simulink model "mip_balance"  (R2017b)
settings: Solver=FixedStepDiscrete  StartTime=0.0  StopTime=inf  RelTol=1e-3  EnableMultiTasking=on
undefined symbols (not defined in the file): DiscIntNeverNeededParam
libraries: beaglebonebluelib x8, simulink_extras x1, simulink x1
settings Model: FPTRunName=Active  SimulationMode=external  ExtModeTrigDuration=2  Creator=The MathWorks, Inc.  LastModifiedBy=pthb3
settings SolverCC: PositivePriorityOrder=on
settings DataIOCC: LimitDataPoints=on  SaveFormat=Array
settings OptimizationCC: ExpressionDepthLimit=2147483647  LifeSpan=Inf  MaxStackSize=64
settings DebuggingCC: UnderspecifiedInitializationDetection=Classic  MergeDetectMultiDrivingBlocksExec=none  FcnCallInpInsideContextMsg=warning  AllowSymbolicDim=off  StateNameClashWarn=warning  SFUnexpectedBacktrackingDiag=warning  SFNoUnconditionalDefaultTransitionDiag=warning  SFExecutionAtInitializationDiag=none
settings HardwareCC: ProdBitPerPointer=32  ProdBitPerSizeT=32  ProdBitPerPtrDiffT=32  ProdLargestAtomicInteger=Long  ProdLargestAtomicFloat=Double  ProdWordSize=32  ProdHWDeviceType=ARM Compatible->ARM Cortex  UseEmbeddedCoderFeatures=off
settings ModelReferenceCC: PropagateSignalLabelsOutOfModel=off
settings RTWCC: SystemTargetFile=ert.tlc  HardwareBoard=BeagleBone Blue  TemplateMakefile=ert_default_tmf  RTWVerbose=off  Toolchain=GNU GCC BeagleBone Blue
settings CodeAppCC: StateflowObjectComments=on
settings ERTTargetCC: MultiwordLength=2048  ERTCustomFileBanners=off  SupportContinuousTime=on  SupportNonInlinedSFcns=on  RemoveResetFunc=off  SupportVariableSizeSignals=on  ModelStepFunctionPrototypeControlCompliant=off  ConvertIfToSwitch=off  SuppressUnreachableDefaultCases=off
settings ConfigComp: CovMetricSettings=dw  CovHtmlReporting=on  CovSaveCumulativeToWorkspaceVar=on  CovSaveSingleToWorkspaceVar=on  CovExternalEMLEnable=off  CovSFcnEnable=off

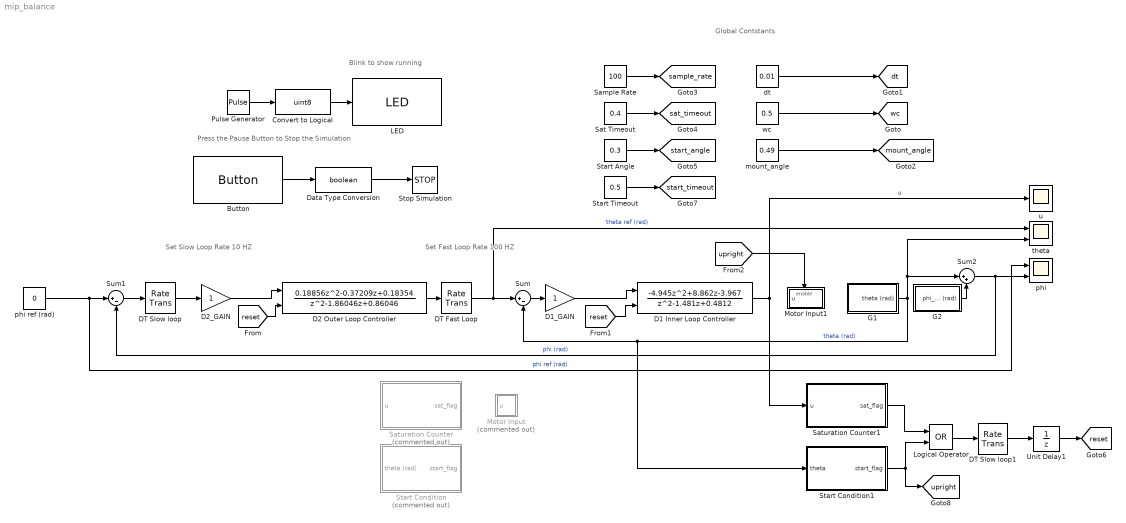
== system mip_balance ==
  note: Global Contstants
  note: Press the Pause Button to Stop the Simulation
  note: Blink to show running
  note: Set Fast Loop Rate
      | 100 HZ
  note: Set Slow Loop Rate
      | 10 HZ
  Button : beaglebonebluelib/Button  Button=Pause  SampleTime=0.1  SimulateUsing=Code generation
      settings: SourceProductName=Simulink Coder Support Package for BeagleBone Blue Hardware
  Convert to Logical : DataTypeConversion  OutDataTypeStr=uint8
  D1 Inner Loop Controller : DiscreteTransferFcn  Numerator=[-4.945, 8.862, -3.967]  Denominator=[1.000, -1.481, 0.4812]  ExternalReset=Rising
      settings: InputPortMap=u0,r7
  D1_GAIN : Gain
  D2 Outer Loop Controller : DiscreteTransferFcn  Numerator="[0.18856,  -0.37209,  0.18354]"  Denominator="[1.00000,  -1.86046,   0.86046]"  ExternalReset=Rising
      settings: InputPortMap=u0,r7
  D2_GAIN : Gain
  DT Fast Loop : RateTransition  OutPortSampleTimeOpt=Multiple of input port sample time  OutPortSampleTimeMultiple=0.1  OutPortSampleTime=0.05
  DT Slow loop : RateTransition  OutPortSampleTime=0.1
  DT Slow loop1 : RateTransition  OutPortSampleTime=0.1
  Data Type Conversion : DataTypeConversion  OutDataTypeStr=boolean
  G1 : Subsystem
  G2 : Subsystem
  LED : beaglebonebluelib/LED  LED=Green
      settings: SourceProductName=Simulink Coder Support Package for BeagleBone Blue Hardware
  Logical Operator : Logic  Operator=OR  AllPortsSameDT=off  OutDataTypeStr=boolean
  Motor Input : Subsystem  Commented=on
  Motor Input1 : Subsystem  TreatAsAtomicUnit=on
  Pulse Generator : DiscretePulseGenerator  Period=10  PulseWidth=5  SampleTime=0.1
  Sample Rate : Constant  Value=100
  Sat Timeout : Constant  Value=0.4
  Saturation Counter : Subsystem  Commented=on
  Saturation Counter1 : Subsystem
  Start Angle : Constant  Value=0.3
  Start Condition : Subsystem  Commented=on
  Start Condition1 : Subsystem
  Start Timeout : Constant  Value=0.5
  Stop Simulation : Stop
  Sum : Sum  Inputs=|+-
  Sum1 : Sum  Inputs=|+-
  Sum2 : Sum  Inputs=|++
  Unit Delay1 : UnitDelay  SampleTime=-1
  dt : Constant  Value=0.01
  mount_angle : Constant  Value=0.49
  phi : Scope  NumInputPorts=2
  phi ref (rad) : Constant  Value=0
  theta : Scope  NumInputPorts=2
  u : Scope
  wc : Constant  Value=0.5
  tag scope: dt=global, mount_angle=global, reset=global, sample_rate=global, sat_timeout=global, start_angle=global, start_timeout=global, upright=global, wc=global
  wires:
  Convert to Logical/1 -> LED/1
  Pulse Generator/1 -> Convert to Logical/1
  Data Type Conversion/1 -> Stop Simulation/1
  Button/1 -> Data Type Conversion/1
  DT Slow loop/1 -> D2_GAIN/1
  wc/1 -> [wc]
  G1/1(theta (rad)) -> theta/2, Sum2/1, Start Condition1/1(theta), Sum/2  "theta (rad)"
  G2/1(phi_enc (rad)) -> Sum2/2
  D2_GAIN/1 -> D2 Outer Loop Controller/1
  Sum/1 -> D1_GAIN/1
  Sum2/1 -> Sum1/2, phi/2  "phi (rad)"
  phi ref (rad)/1 -> phi/1, Sum1/1  "phi ref (rad)"
  dt/1 -> [dt]
  D1 Inner Loop Controller/1 -> Saturation Counter1/1(u), u/1  "u"
  D1_GAIN/1 -> D1 Inner Loop Controller/1
  D2 Outer Loop Controller/1 -> DT Fast Loop/1
  Sum1/1 -> DT Slow loop/1
  DT Fast Loop/1 -> theta/1, Sum/1  "theta ref (rad)"
  mount_angle/1 -> [mount_angle]
  Sample Rate/1 -> [sample_rate]
  Start Angle/1 -> [start_angle]
  Sat Timeout/1 -> [sat_timeout]
  Start Condition1/1(start_flag) -> [upright], Logical Operator/2
  Saturation Counter1/1(sat_flag) -> Logical Operator/1
  Logical Operator/1 -> DT Slow loop1/1
  [reset] -> D1 Inner Loop Controller/2
  [reset] -> D2 Outer Loop Controller/2
  Unit Delay1/1 -> [reset]
  DT Slow loop1/1 -> Unit Delay1/1
  Start Timeout/1 -> [start_timeout]
  [upright] -> Motor Input1/Enable

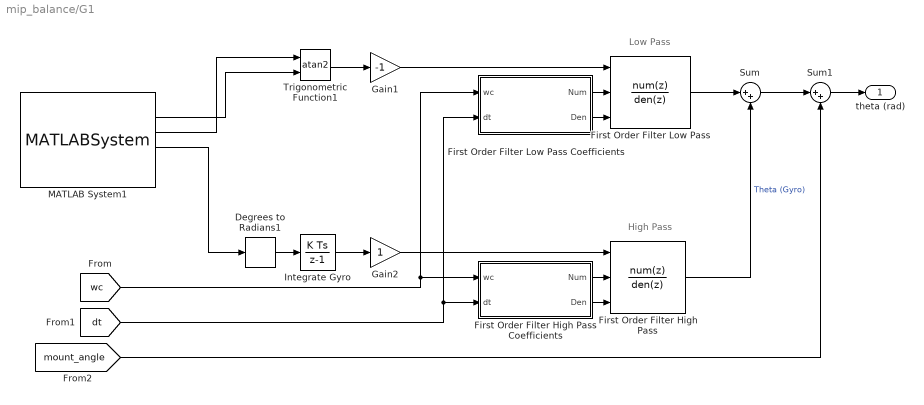
== system mip_balance/G1 ==
  note: High Pass
  note: Low Pass
  Degrees to Radians1 : simulink_extras/Transformations/Degrees to Radians
  First Order Filter High Pass : DiscreteTransferFcn  NumeratorSource=Input port  DenominatorSource=Input port  Denominator=[1]  a0EqualsOne=on
      settings: InputPortMap=u0,p1,p3
  First Order Filter High Pass Coefficients : MATLAB Function  TreatAsAtomicUnit=on
  First Order Filter Low Pass : DiscreteTransferFcn  NumeratorSource=Input port  DenominatorSource=Input port  Denominator=[1]  a0EqualsOne=on
      settings: InputPortMap=u0,p1,p3
  First Order Filter Low Pass Coefficients : MATLAB Function  TreatAsAtomicUnit=on
  Gain1 : Gain  Gain=-1
  Gain2 : Gain
  Integrate Gyro : DiscreteIntegrator  InitialConditionSetting=State (most efficient)  SampleTime=-1  ICPrevOutput=DiscIntNeverNeededParam  ICPrevScaledInput=DiscIntNeverNeededParam
  MATLAB System1 : MATLABSystem  System=beagleboneblue.fccr_bbblueIMU  SampleTime=0.01
      mask Type: beagleboneblue.fccr_bbblueIMU
      mask Display:
      | color('white');
      | plot([100,100,100,100]*1,[100,100,100,100]*1);
      | plot([100,100,100,100]*0,[100,100,100,100]*0);
      | color('blue');
      | text(100, 92, ' BB BLUE ', 'horizontalAlignment', 'right');
      | color('black');
      | text(52,52,' IMU','horizontalAlignment','center');
      | color('black');
  Sum : Sum  Inputs=|++
  Sum1 : Sum  Inputs=|++
  Trigonometric Function1 : Trigonometry  Operator=atan2
  theta (rad) : Outport
  wires:
  First Order Filter Low Pass Coefficients/1(Num) -> First Order Filter Low Pass/2
  Gain2/1 -> First Order Filter High Pass/1
  First Order Filter Low Pass Coefficients/2(Den) -> First Order Filter Low Pass/3
  MATLAB System1/4 -> Degrees to Radians1/1
  Trigonometric Function1/1 -> Gain1/1
  [wc] -> First Order Filter Low Pass Coefficients/1(wc), First Order Filter High Pass Coefficients/1(wc)
  [dt] -> First Order Filter Low Pass Coefficients/2(dt), First Order Filter High Pass Coefficients/2(dt)
  First Order Filter High Pass Coefficients/2(Den) -> First Order Filter High Pass/3
  First Order Filter Low Pass/1 -> Sum/1
  Gain1/1 -> First Order Filter Low Pass/1
  Integrate Gyro/1 -> Gain2/1
  First Order Filter High Pass/1 -> Sum/2  "Theta (Gyro)"
  Degrees to Radians1/1 -> Integrate Gyro/1
  Sum/1 -> Sum1/1
  MATLAB System1/2 -> Trigonometric Function1/2
  First Order Filter High Pass Coefficients/1(Num) -> First Order Filter High Pass/2
  MATLAB System1/3 -> Trigonometric Function1/1
  Sum1/1 -> theta (rad)/1
  [mount_angle] -> Sum1/2

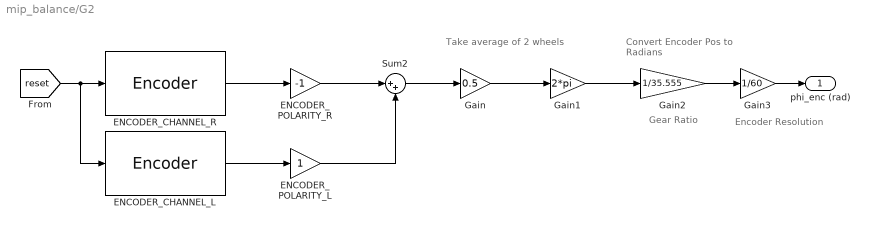
== system mip_balance/G2 ==
  note: Encoder
      | Resolution
  note: Gear Ratio
  note: Convert Encoder Pos
      | to Radians
  note: Take average
      | of 2 wheels
  ENCODER_CHANNEL_L : beaglebonebluelib/Encoder  Channel=3  Mode=Reset by external signal  SampleTime=0.01  SimulateUsing=Code generation
      settings: SourceProductName=Simulink Coder Support Package for BeagleBone Blue Hardware
  ENCODER_CHANNEL_R : beaglebonebluelib/Encoder  Channel=2  Mode=Reset by external signal  SampleTime=0.01  SimulateUsing=Code generation
      settings: SourceProductName=Simulink Coder Support Package for BeagleBone Blue Hardware
  ENCODER_POLARITY_L : Gain
  ENCODER_POLARITY_R : Gain  Gain=-1
  Gain : Gain  Gain=0.5  OutDataTypeStr=double
  Gain1 : Gain  Gain=2*pi
  Gain2 : Gain  Gain=1/35.555
  Gain3 : Gain  Gain=1/60
  Sum2 : Sum  Inputs=|++
  phi_enc (rad) : Outport
  wires:
  ENCODER_POLARITY_R/1 -> Sum2/1
  ENCODER_POLARITY_L/1 -> Sum2/2
  ENCODER_CHANNEL_L/1 -> ENCODER_POLARITY_L/1
  ENCODER_CHANNEL_R/1 -> ENCODER_POLARITY_R/1
  Sum2/1 -> Gain/1
  Gain/1 -> Gain1/1
  Gain1/1 -> Gain2/1
  Gain2/1 -> Gain3/1
  Gain3/1 -> phi_enc (rad)/1
  [reset] -> ENCODER_CHANNEL_L/1, ENCODER_CHANNEL_R/1

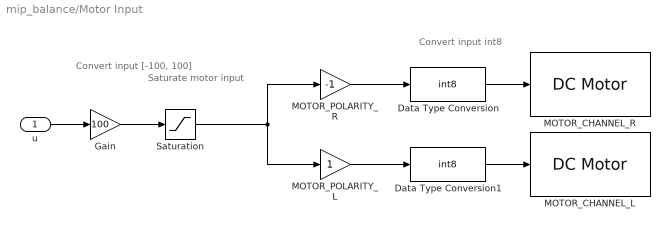
== system mip_balance/Motor Input ==
  note: Saturate motor
      | input
  note: Convert input
      | int8
  note: Convert input
      | [-100, 100]
  u : Inport
  Data Type Conversion : DataTypeConversion  OutDataTypeStr=int8  SaturateOnIntegerOverflow=on  RndMeth=Zero
  Data Type Conversion1 : DataTypeConversion  OutDataTypeStr=int8  SaturateOnIntegerOverflow=on  RndMeth=Zero
  Gain : Gain  Gain=100
  MOTOR_CHANNEL_L : beaglebonebluelib/DC Motor  index=3  stopaction=Free Spin  SimulateUsing=Code generation
      settings: SourceProductName=Simulink Coder Support Package for BeagleBone Blue Hardware
  MOTOR_CHANNEL_R : beaglebonebluelib/DC Motor  index=2  stopaction=Free Spin  SimulateUsing=Code generation
      settings: SourceProductName=Simulink Coder Support Package for BeagleBone Blue Hardware
  MOTOR_POLARITY_L : Gain
  MOTOR_POLARITY_R : Gain  Gain=-1
  Saturation : Saturate  UpperLimit=100  LowerLimit=-100  RndMeth=Zero
  wires:
  u/1 -> Gain/1
  Gain/1 -> Saturation/1
  MOTOR_POLARITY_R/1 -> Data Type Conversion/1
  MOTOR_POLARITY_L/1 -> Data Type Conversion1/1
  Saturation/1 -> MOTOR_POLARITY_R/1, MOTOR_POLARITY_L/1
  Data Type Conversion/1 -> MOTOR_CHANNEL_R/1
  Data Type Conversion1/1 -> MOTOR_CHANNEL_L/1

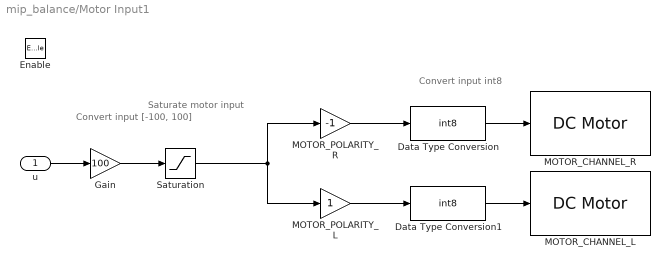
== system mip_balance/Motor Input1 ==
  note: Convert input
      | [-100, 100]
  note: Convert input
      | int8
  note: Saturate motor
      | input
  u : Inport
  Enable : EnablePort  StatesWhenEnabling=reset
  Data Type Conversion : DataTypeConversion  OutDataTypeStr=int8  SaturateOnIntegerOverflow=on  RndMeth=Zero
  Data Type Conversion1 : DataTypeConversion  OutDataTypeStr=int8  SaturateOnIntegerOverflow=on  RndMeth=Zero
  Gain : Gain  Gain=100
  MOTOR_CHANNEL_L : beaglebonebluelib/DC Motor  index=3  stopaction=Free Spin  SimulateUsing=Code generation
      settings: SourceProductName=Simulink Coder Support Package for BeagleBone Blue Hardware
  MOTOR_CHANNEL_R : beaglebonebluelib/DC Motor  index=2  stopaction=Free Spin  SimulateUsing=Code generation
      settings: SourceProductName=Simulink Coder Support Package for BeagleBone Blue Hardware
  MOTOR_POLARITY_L : Gain
  MOTOR_POLARITY_R : Gain  Gain=-1
  Saturation : Saturate  UpperLimit=100  LowerLimit=-100  RndMeth=Zero
  wires:
  MOTOR_POLARITY_R/1 -> Data Type Conversion/1
  MOTOR_POLARITY_L/1 -> Data Type Conversion1/1
  u/1 -> Gain/1
  Gain/1 -> Saturation/1
  Saturation/1 -> MOTOR_POLARITY_R/1, MOTOR_POLARITY_L/1
  Data Type Conversion/1 -> MOTOR_CHANNEL_R/1
  Data Type Conversion1/1 -> MOTOR_CHANNEL_L/1

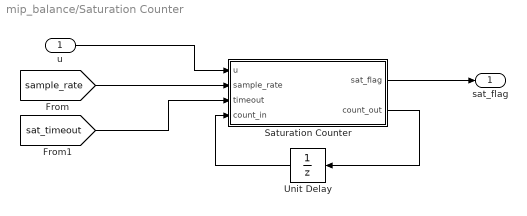
== system mip_balance/Saturation Counter ==
  u : Inport
  Saturation Counter : MATLAB Function  TreatAsAtomicUnit=on
  Unit Delay : UnitDelay  SampleTime=-1
  sat_flag : Outport
  wires:
  Saturation Counter/2(count_out) -> Unit Delay/1
  Unit Delay/1 -> Saturation Counter/4(count_in)
  u/1 -> Saturation Counter/1(u)
  [sat_timeout] -> Saturation Counter/3(timeout)
  [sample_rate] -> Saturation Counter/2(sample_rate)
  Saturation Counter/1(sat_flag) -> sat_flag/1

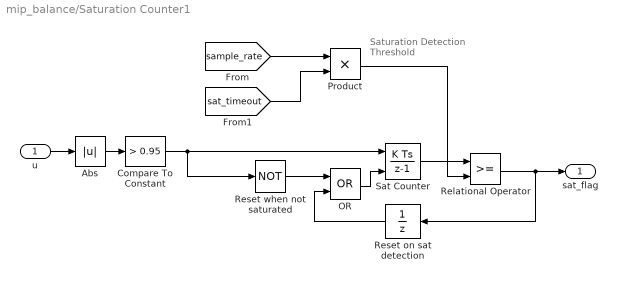
== system mip_balance/Saturation Counter1 ==
  note: Saturation Detection
      | Threshold
  u : Inport
  Abs : Abs
  Compare To Constant : simulink/Logic and Bit Operations/Compare To Constant  relop=>  const=0.95  OutDataTypeStr=boolean
  OR : Logic  Operator=OR  AllPortsSameDT=off  OutDataTypeStr=boolean
  Product : Product
  Relational Operator : RelationalOperator  OutDataTypeStr=boolean  RndMeth=Simplest
  Reset on sat detection : UnitDelay  SampleTime=-1
  Reset when not saturated : Logic  Operator=NOT  AllPortsSameDT=off  OutDataTypeStr=boolean
  Sat Counter : DiscreteIntegrator  ExternalReset=rising  InitialConditionSetting=State (most efficient)  SampleTime=-1  ICPrevOutput=DiscIntNeverNeededParam  ICPrevScaledInput=DiscIntNeverNeededParam
  sat_flag : Outport
  wires:
  u/1 -> Abs/1
  Sat Counter/1 -> Relational Operator/1
  Relational Operator/1 -> sat_flag/1, Reset on sat detection/1
  Compare To Constant/1 -> Reset when not saturated/1, Sat Counter/1
  Abs/1 -> Compare To Constant/1
  [sample_rate] -> Product/1
  [sat_timeout] -> Product/2
  Product/1 -> Relational Operator/2
  OR/1 -> Sat Counter/2
  Reset on sat detection/1 -> OR/2
  Reset when not saturated/1 -> OR/1

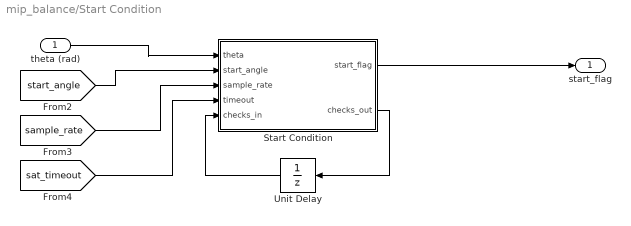
== system mip_balance/Start Condition ==
  theta (rad) : Inport
  Start Condition : MATLAB Function  TreatAsAtomicUnit=on
  Unit Delay : UnitDelay  SampleTime=-1
  start_flag : Outport
  wires:
  Start Condition/1(start_flag) -> start_flag/1
  Unit Delay/1 -> Start Condition/5(checks_in)
  Start Condition/2(checks_out) -> Unit Delay/1
  [sat_timeout] -> Start Condition/4(timeout)
  [sample_rate] -> Start Condition/3(sample_rate)
  theta (rad)/1 -> Start Condition/1(theta)
  [start_angle] -> Start Condition/2(start_angle)

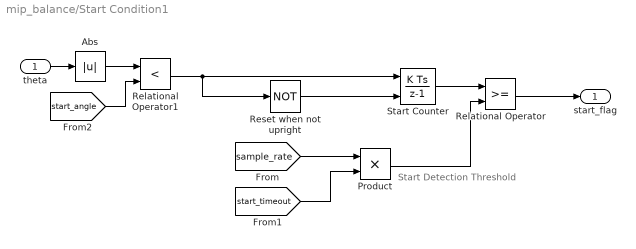
== system mip_balance/Start Condition1 ==
  note: Start Detection
      | Threshold
  theta : Inport
  Abs : Abs
  Product : Product
  Relational Operator : RelationalOperator  OutDataTypeStr=boolean  RndMeth=Simplest
  Relational Operator1 : RelationalOperator  Operator=<  OutDataTypeStr=boolean  RndMeth=Simplest
  Reset when not upright : Logic  Operator=NOT  AllPortsSameDT=off  OutDataTypeStr=boolean
  Start Counter : DiscreteIntegrator  ExternalReset=rising  InitialConditionSetting=State (most efficient)  SampleTime=-1  ICPrevOutput=DiscIntNeverNeededParam  ICPrevScaledInput=DiscIntNeverNeededParam
  start_flag : Outport
  wires:
  theta/1 -> Abs/1
  Start Counter/1 -> Relational Operator/1
  Relational Operator/1 -> start_flag/1
  Relational Operator1/1 -> Reset when not upright/1, Start Counter/1
  Abs/1 -> Relational Operator1/1
  [sample_rate] -> Product/1
  [start_timeout] -> Product/2
  Product/1 -> Relational Operator/2
  Reset when not upright/1 -> Start Counter/2
  [start_angle] -> Relational Operator1/2

== matlab function mip_balance/G1/First Order Filter High Pass Coefficients ==
  data: wc input; Num output; dt input; Den output
function [Num, Den] = first_order_hp(wc,dt)
%#codegen
Num = [1 -1];
Den = [1 (wc*dt - 1)];

== matlab function mip_balance/G1/First Order Filter Low Pass Coefficients ==
  data: wc input; Num output; dt input; Den output
function [Num, Den] = first_order_lp(wc,dt)
%#codegen
Num = [0 wc*dt];
Den = [1 (wc*dt - 1)];

== matlab function mip_balance/Saturation Counter/Saturation Counter ==
  data: sat_flag output; u input; sample_rate input; timeout input; count_out output; count_in input
function [sat_flag, count_out] = sat_counter(u, sample_rate, timeout, count_in)

if abs(u) > 0.95
    count_in = count_in + 1;
else
    count_in = 0;
end

if count_in > (sample_rate*timeout)
    sat_flag = 1;
%     count_in = 0;
else
    sat_flag = 0;
end

count_out = count_in;
end

== matlab function mip_balance/Start Condition/Start Condition ==
  data: theta input; start_angle input; start_flag output; sample_rate input; timeout input; checks_in input; checks_out output
function [start_flag, checks_out] = start_condition(theta, start_angle, sample_rate, timeout, checks_in)

start_flag = 0;

if abs(theta) < start_angle
    checks_in = checks_in + 1;
else
    checks_in = 0;
end

if checks_in > (sample_rate*timeout)
    start_flag = 1;
end

checks_out = checks_in;
end
